simulink model "idle_speed_model_project_pid"  (Simulink 9.1)
settings: Solver=ode45  StartTime=0  StopTime=25  FixedStep=0.01  MaxStep=0.02  RelTol=1e-3  EnableMultiTasking=on
values from neighbouring files (symbols this model uses):
  a = [1.69e-07,-1.136e-06,6.89e-06]    [assign_pid.m]
  gam = 1.35    [assign_pid.m]
  J = 0.0789    [assign_pid.m]
  Kd = 4    [assign_pid.m]
  KI = 0.005    [assign_pid.m]
  KP = 0.8    [assign_pid.m]
  N0 = 828    [assign_pid.m]
  P0 = 26431    [assign_pid.m]
  p_amb = 1.0121*1e5    (= 101210)    [assign_pid.m]
  par_fr = [7.4198e-7 -4.989e-4 11.3]    [assign_pid.m]
  par_IMEP0 = [1.2323e-4 2.1256]    [assign_pid.m]
  par_sp = [-0.0017 -0.0277 1.36]    [assign_pid.m]
  R = 288    [assign_pid.m]
  si = 0.812    [assign_pid.m]
  T_amb = 302    [assign_pid.m]
  Tau_d = pi/3    (= 1.0471975512)    [assign_pid.m]
  Vd = 2.4e-3    (= 0.0024)    [assign_pid.m]
  Vm = 5.8e-3    (= 0.0058)    [assign_pid.m]
  X0 = [26424 21.3765773202354 83.9019428270409]    [assign_pid.m]
  yi = 0.0633    [assign_pid.m]
  Z = 4    [assign_pid.m]
undefined symbols (not defined in the file or in its folder): setp, sigbuilder_block
settings Model: Creator=Canov  LastModifiedBy=VARUN
settings SolverCC: PositivePriorityOrder=on
settings DataIOCC: SignalLoggingSaveFormat=ModelDataLogs  SignalLoggingName=sigsOut
settings OptimizationCC: ExpressionDepthLimit=2147483647  InitFltsAndDblsToZero=on
settings DebuggingCC: SaveWithParameterizedLinksMsg=none  SignalResolutionControl=TryResolveAllWithWarning  MultiTaskDSMMsg=warning  MultiTaskCondExecSysMsg=none  FcnCallInpInsideContextMsg=warning  StateNameClashWarn=warning
settings HardwareCC: TargetBitPerPointer=64  TargetBitPerSizeT=64  TargetBitPerPtrDiffT=64  TargetLongLongMode=on  TargetIntDivRoundTo=Zero  TargetEndianess=LittleEndian  TargetWordSize=64  TargetHWDeviceType=MATLAB Host  ProdEqTarget=off
settings GRTTargetCC: TargetFcnLib=ansi_tfl_tmw.mat  GeneratePreprocessorConditionals=Disable all

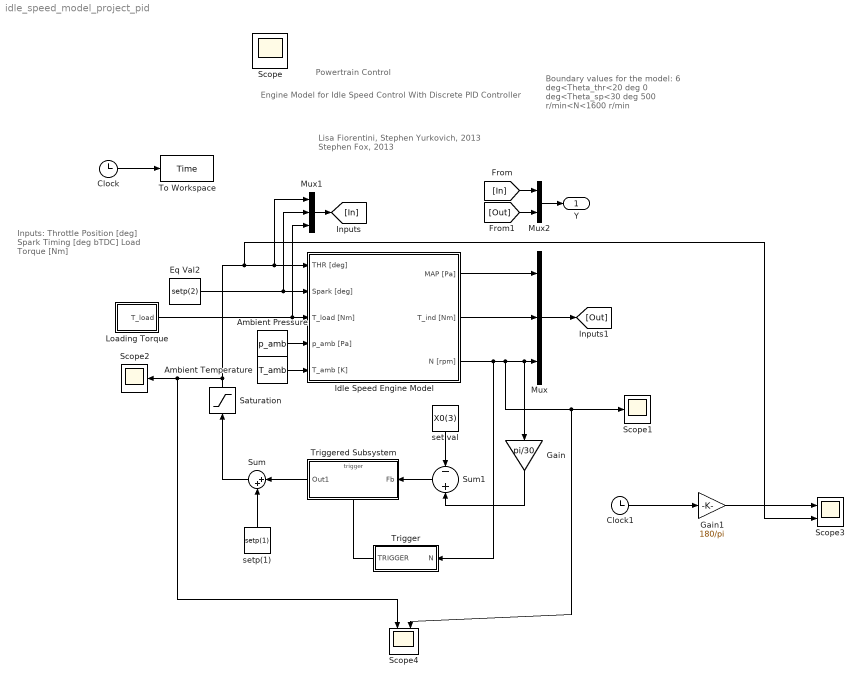
== system idle_speed_model_project_pid ==
  note: Engine Model for Idle Speed Control
      | With Discrete PID Controller
  note: Inputs:
      |
      |
      | Throttle Position [deg]
      |
      | Spark Timing [deg bTDC]
      |
      | Load Torque [Nm]
  note: Powertrain Control
  note: Lisa Fiorentini, Stephen Yurkovich, 2013
      | Stephen Fox, 2013
  note: Boundary values for the model:
      | 6 deg<Theta_thr<20 deg
      | 0 deg<Theta_sp<30 deg
      | 500 r/min<N<1600 r/min
  Ambient Pressure : Constant  Value=p_amb
  Ambient Temperature : Constant  Value=T_amb
  Clock : Clock
  Clock1 : Clock
  Eq Val2 : Constant  Value=setp(2)
  Gain : Gain  Gain=pi/30
  Gain1 : Gain  Gain=180/pi
  Idle Speed Engine Model : Subsystem
  Loading Torque : Subsystem
  Mux : Mux  Inputs=3
  Mux1 : Mux  Inputs=3
  Mux2 : Mux  Inputs=2
  Saturation : Saturate  UpperLimit=20  LowerLimit=6  OutMin=[6]  OutMax=[20]
  Scope1 : Scope
  Scope2 : Scope
  Scope3 : Scope  NumInputPorts=2
  Scope4 : Scope  NumInputPorts=2
  Sum : Sum  Inputs=|++
  Sum1 : Sum  Inputs=-|+
  To Workspace : ToWorkspace  VariableName=Time  SaveFormat=Structure  SampleTime=-1
      settings: Decimation=7  Save2DSignal=2-D array (concatenate along first dimension)
  Trigger : Subsystem
  Triggered Subsystem : Subsystem  TreatAsAtomicUnit=on
  set val : Constant  Value=X0(3)
  setp(1) : Constant  Value=setp(1)
  Y : Outport
  Scope : Scope
  wires:
  Ambient Pressure/1 -> Idle Speed Engine Model/4(p_amb [Pa])
  Ambient Temperature/1 -> Idle Speed Engine Model/5(T_amb [K])
  Eq Val2/1 -> Idle Speed Engine Model/2(Spark [deg]), Mux1/2
  Idle Speed Engine Model/2(T_ind [Nm]) -> Mux/2
  Idle Speed Engine Model/1(MAP [Pa]) -> Mux/1
  Loading Torque/1(T_load) -> Idle Speed Engine Model/3(T_load [Nm]), Mux1/3
  Idle Speed Engine Model/3(N [rpm]) -> Trigger/1(N), Scope4/2, Scope1/1, Mux/3, Gain/1
  Sum/1 -> Saturation/1
  Mux1/1 -> [In]
  Mux/1 -> [Out]
  [In] -> Mux2/1
  [Out] -> Mux2/2
  Mux2/1 -> Y/1
  Triggered Subsystem/1(Out1) -> Sum/1
  setp(1)/1 -> Sum/2
  Gain/1 -> Sum1/2
  Sum1/1 -> Triggered Subsystem/1(Fb)
  set val/1 -> Sum1/1
  Saturation/1 -> Scope4/1, Scope2/1, Scope3/2, Idle Speed Engine Model/1(THR [deg]), Mux1/1
  Trigger/1(TRIGGER) -> Triggered Subsystem/Trigger
  Clock/1 -> To Workspace/1
  Clock1/1 -> Gain1/1
  Gain1/1 -> Scope3/1

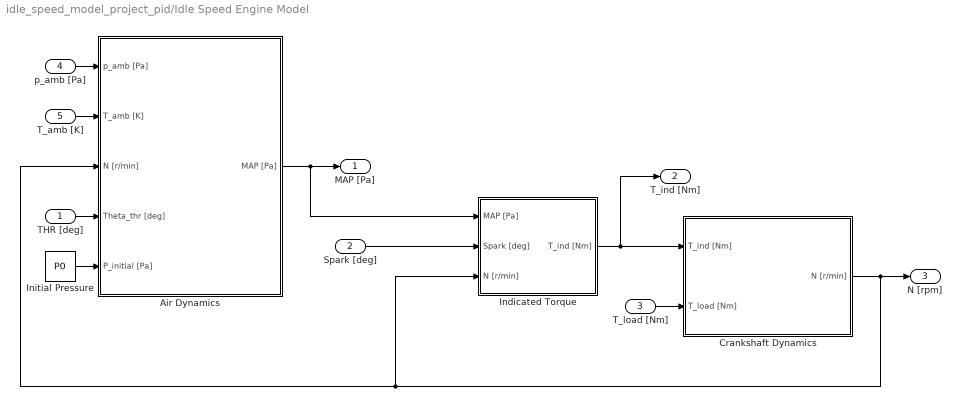
== system idle_speed_model_project_pid/Idle Speed Engine Model ==
  THR [deg] : Inport
  Spark [deg] : Inport  Port=2
  T_load [Nm] : Inport  Port=3
  p_amb [Pa] : Inport  Port=4
  T_amb [K] : Inport  Port=5
  Air Dynamics : Subsystem
  Crankshaft Dynamics : Subsystem
  Indicated Torque : Subsystem
  Initial Pressure : Constant  Value=P0
  MAP [Pa] : Outport
  T_ind [Nm] : Outport  Port=2
  N [rpm] : Outport  Port=3
  wires:
  Spark [deg]/1 -> Indicated Torque/2(Spark [deg])
  Indicated Torque/1(T_ind [Nm]) -> T_ind [Nm]/1, Crankshaft Dynamics/1(T_ind [Nm])
  Air Dynamics/1(MAP [Pa]) -> Indicated Torque/1(MAP [Pa]), MAP [Pa]/1
  Crankshaft Dynamics/1(N [r/min]) -> Indicated Torque/3(N [r/min]), Air Dynamics/3(N [r/min]), N [rpm]/1
  p_amb [Pa]/1 -> Air Dynamics/1(p_amb [Pa])
  T_amb [K]/1 -> Air Dynamics/2(T_amb [K])
  THR [deg]/1 -> Air Dynamics/4(Theta_thr [deg])
  Initial Pressure/1 -> Air Dynamics/5(P_initial [Pa])
  T_load [Nm]/1 -> Crankshaft Dynamics/2(T_load [Nm])

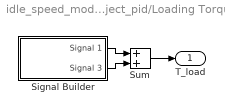
== system idle_speed_model_project_pid/Loading Torque ==
  Signal Builder : Subsystem  Tag=STV Subsys  LoadFcn=sigbuilder_block('load');  StartFcn=sigbuilder_block('start');  StopFcn=sigbuilder_block('stop');  ClipboardFcn=sigbuilder_block('clipboard');  mask(Sigbuilder block){tuvar=[0:10]}
      mask help: Simulink:masks:SigbuilderBlock_MD
      mask init:
      | if ~strcmp(get_param(bdroot(gcbh),'SimulationStatus'),'stopped') tuvar = sigbuilder_block('maskInit'); end
      settings: CopyFcn=sigbuilder_block('copy');  DeleteFcn=sigbuilder_block('delete');  ModelCloseFcn=sigbuilder_block('modelClose');  PreSaveFcn=sigbuilder_block('preSave');  PauseFcn=sigbuilder_block('pause');  ContinueFcn=sigbuilder_block('continue');  NameChangeFcn=sigbuilder_block('namechange');  OpenFcn=sigbuilder_block('open',[6 30 1012.5 447.75 ]);  CloseFcn=sigbuilder_block('close');
      mask Display: plot(0, 0, 100, 100,[2, 2, 32, 32, 2], [68, 8, 8, 68, 68],[32, 2], [38, 38], [32, 19, 2],[53, 60, 44], [32, 17, 17, 2],[16, 16, 31, 31]);txt = getActiveGroup(gcbh);text(2, 100, txt,'verticalAlignment', 'top');
  Sum : Sum
  T_load : Outport
  wires:
  Signal Builder/1(Signal 1) -> Sum/1
  Signal Builder/2(Signal 3) -> Sum/2
  Sum/1 -> T_load/1

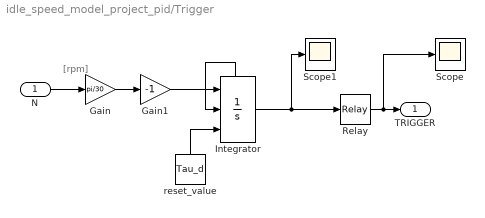
== system idle_speed_model_project_pid/Trigger ==
  note: [rpm]
  N : Inport
  Gain : Gain  Gain=pi/30
  Gain1 : Gain  Gain=-1
  Integrator : Integrator  ExternalReset=falling  InitialConditionSource=external  ShowStatePort=on
  Relay : Relay  OnSwitchValue=0.5*Tau_d  OffSwitchValue=0.5*Tau_d
  Scope : Scope
  Scope1 : Scope
  reset_value : Constant  Value=Tau_d
  TRIGGER : Outport
  wires:
  Relay/1 -> Scope/1, TRIGGER/1
  reset_value/1 -> Integrator/3
  Gain1/1 -> Integrator/1
  Integrator/State -> Integrator/2
  N/1 -> Gain/1
  Gain/1 -> Gain1/1
  Integrator/1 -> Scope1/1, Relay/1

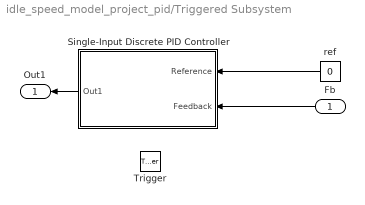
== system idle_speed_model_project_pid/Triggered Subsystem ==
  Fb : Inport
  Trigger : TriggerPort  VariantControl=Variant  PortDimensions=1
  Single-Input Discrete PID Controller : Subsystem
  ref : Constant  Value=0
  Out1 : Outport
  wires:
  ref/1 -> Single-Input Discrete PID Controller/1(Reference)
  Single-Input Discrete PID Controller/1(Out1) -> Out1/1
  Fb/1 -> Single-Input Discrete PID Controller/2(Feedback)

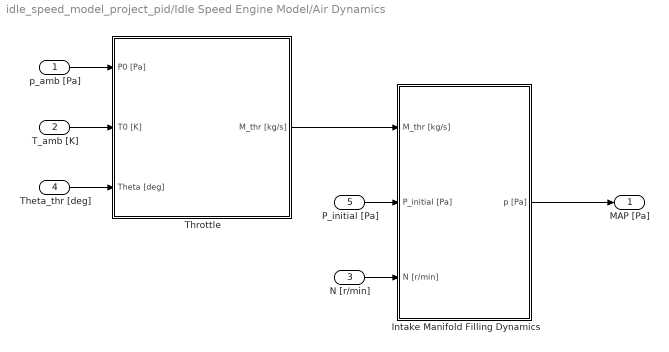
== system idle_speed_model_project_pid/Idle Speed Engine Model/Air Dynamics ==
  p_amb [Pa] : Inport
  T_amb [K] : Inport  Port=2
  N [r/min] : Inport  Port=3
  Theta_thr [deg] : Inport  Port=4
  P_initial [Pa] : Inport  Port=5
  Intake Manifold Filling Dynamics : Subsystem
  Throttle : Subsystem
  MAP [Pa] : Outport
  wires:
  Intake Manifold Filling Dynamics/1(p [Pa]) -> MAP [Pa]/1
  P_initial [Pa]/1 -> Intake Manifold Filling Dynamics/2(P_initial [Pa])
  p_amb [Pa]/1 -> Throttle/1(P0 [Pa])
  T_amb [K]/1 -> Throttle/2(T0 [K])
  Theta_thr [deg]/1 -> Throttle/3(Theta [deg])
  Throttle/1(M_thr [kg/s]) -> Intake Manifold Filling Dynamics/1(M_thr [kg/s])
  N [r/min]/1 -> Intake Manifold Filling Dynamics/3(N [r/min])

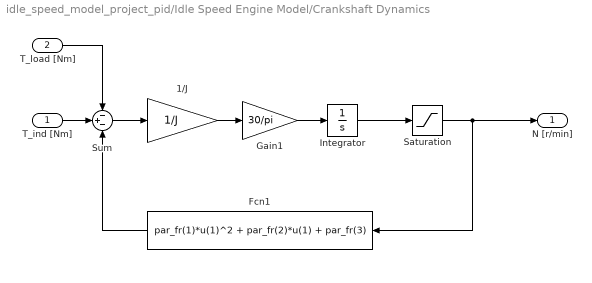
== system idle_speed_model_project_pid/Idle Speed Engine Model/Crankshaft Dynamics ==
  T_ind [Nm] : Inport
  T_load [Nm] : Inport  Port=2
  1/J : Gain  Gain=1/J  SaturateOnIntegerOverflow=on  OutDataTypeStr=Inherit: Same as input  ParamDataTypeStr=Inherit: Same as input
  Fcn1 : Fcn  Expr=par_fr(1)*u(1)^2 + par_fr(2)*u(1) + par_fr(3)
  Gain1 : Gain  Gain=30/pi  SaturateOnIntegerOverflow=on  OutDataTypeStr=Inherit: Same as input  ParamDataTypeStr=Inherit: Same as input
  Integrator : Integrator  InitialCondition=N0
  Saturation : Saturate  UpperLimit=6000  LowerLimit=100
  Sum : Sum  Inputs=-+-  SaturateOnIntegerOverflow=on
  N [r/min] : Outport
  wires:
  Saturation/1 -> N [r/min]/1, Fcn1/1
  T_ind [Nm]/1 -> Sum/2
  T_load [Nm]/1 -> Sum/1
  Sum/1 -> 1/J/1
  1/J/1 -> Gain1/1
  Gain1/1 -> Integrator/1
  Integrator/1 -> Saturation/1
  Fcn1/1 -> Sum/3

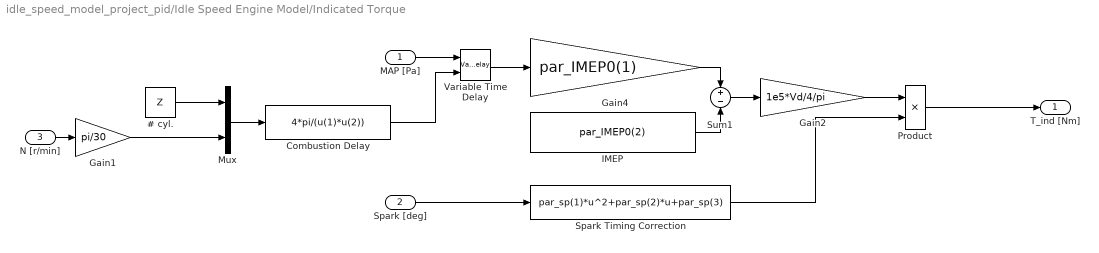
== system idle_speed_model_project_pid/Idle Speed Engine Model/Indicated Torque ==
  MAP [Pa] : Inport
  Spark [deg] : Inport  Port=2
  N [r/min] : Inport  Port=3
  # cyl. : Constant  Value=Z
  Combustion Delay : Fcn  Expr=4*pi/(u(1)*u(2))
  Gain1 : Gain  Gain=pi/30  SaturateOnIntegerOverflow=on  OutDataTypeStr=Inherit: Same as input  ParamDataTypeStr=Inherit: Same as input
  Gain2 : Gain  Gain=1e5*Vd/4/pi  SaturateOnIntegerOverflow=on  OutDataTypeStr=Inherit: Same as input  ParamDataTypeStr=Inherit: Same as input
  Gain4 : Gain  Gain=par_IMEP0(1)  SaturateOnIntegerOverflow=on  OutDataTypeStr=Inherit: Same as input  ParamDataTypeStr=Inherit: Same as input
  IMEP : Constant  Value=par_IMEP0(2)
  Mux : Mux  Inputs=2
  Product : Product  RndMeth=Zero
  Spark Timing Correction : Fcn  Expr=par_sp(1)*u^2+par_sp(2)*u+par_sp(3)
  Sum1 : Sum  Inputs=+-  SaturateOnIntegerOverflow=on
  Variable Time Delay : VariableTransportDelay  InitialOutput=P0  ZeroDelay=on
  T_ind [Nm] : Outport
  wires:
  Spark Timing Correction/1 -> Product/2
  Spark [deg]/1 -> Spark Timing Correction/1
  Gain2/1 -> Product/1
  Gain1/1 -> Mux/2
  Mux/1 -> Combustion Delay/1
  # cyl./1 -> Mux/1
  N [r/min]/1 -> Gain1/1
  Product/1 -> T_ind [Nm]/1
  Gain4/1 -> Sum1/1
  IMEP/1 -> Sum1/2
  Sum1/1 -> Gain2/1
  Combustion Delay/1 -> Variable Time Delay/2
  MAP [Pa]/1 -> Variable Time Delay/1
  Variable Time Delay/1 -> Gain4/1

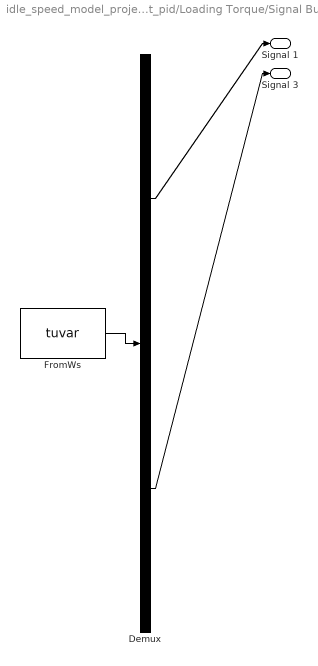
== system idle_speed_model_project_pid/Loading Torque/Signal Builder ==
  Demux : Demux  Tag=STV Demux  Outputs=2
  FromWs : FromWorkspace  Tag=STV FromWs  VariableName=tuvar  SampleTime=0  SigBuilderData=DataTag0  VnvData=DataTag1
      SigBuilderData=|
      | common.afterFinalStr = 'Extrapolate'
      | common.sampleTime = 0
      | dataSet.timeRange = [0 2000]
      | dataSet.name = 'Group 1'
      | sbobj.Groups.Name = 'Group 1'
      | sbobj.Groups.Signals(1).Name = 'Signal 1'
      | sbobj.Groups.Signals(1).XData = [0 5 5 10 10 2000]
      | sbobj.Groups.Signals(1).YData = [10 10 20 20 10 10]
      | sbobj.Groups.Signals(2).Name = 'Signal 3'
      | sbobj.Groups.Signals(2).XData = [0 15 15 20 20 2000]
      | sbobj.Groups.Signals(2).YData = [0 0 -10 -10 0 0]
      | sbobj.Groups.TimeRange = [0 2000]
  Signal 1 : Outport  Tag=STV Outport
  Signal 3 : Outport  Tag=STV Outport  Port=2
  wires:
  FromWs/1 -> Demux/1
  Demux/1 -> Signal 1/1
  Demux/2 -> Signal 3/1

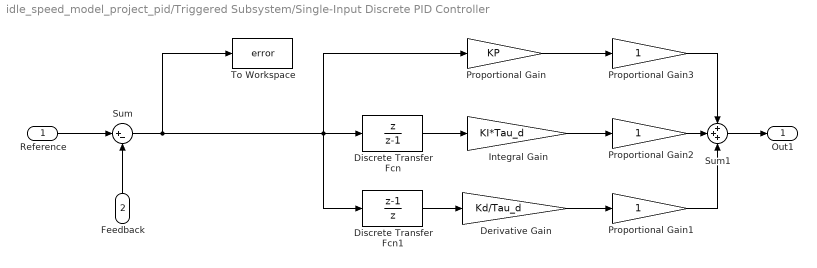
== system idle_speed_model_project_pid/Triggered Subsystem/Single-Input Discrete PID Controller ==
  Reference : Inport
  Feedback : Inport  Port=2
  Derivative Gain : Gain  Gain=Kd/Tau_d
  Discrete Transfer Fcn : DiscreteTransferFcn  Numerator=[1 0]  Denominator=[1 -1]
  Discrete Transfer Fcn1 : DiscreteTransferFcn  Numerator=[1 -1]  Denominator=[1 0]
  Integral Gain : Gain  Gain=KI*Tau_d
  Proportional Gain : Gain  Gain=KP
  Proportional Gain1 : Gain
  Proportional Gain2 : Gain
  Proportional Gain3 : Gain
  Sum : Sum  Inputs=|+-
  Sum1 : Sum  Inputs=+++
  To Workspace : ToWorkspace  VariableName=error  SaveFormat=Structure With Time  SampleTime=-1
      settings: Save2DSignal=2-D array (concatenate along first dimension)
  Out1 : Outport
  wires:
  Discrete Transfer Fcn1/1 -> Derivative Gain/1
  Discrete Transfer Fcn/1 -> Integral Gain/1
  Reference/1 -> Sum/1
  Feedback/1 -> Sum/2
  Proportional Gain/1 -> Proportional Gain3/1
  Integral Gain/1 -> Proportional Gain2/1
  Derivative Gain/1 -> Proportional Gain1/1
  Proportional Gain3/1 -> Sum1/1
  Proportional Gain2/1 -> Sum1/2
  Proportional Gain1/1 -> Sum1/3
  Sum1/1 -> Out1/1
  Sum/1 -> To Workspace/1, Discrete Transfer Fcn1/1, Proportional Gain/1, Discrete Transfer Fcn/1

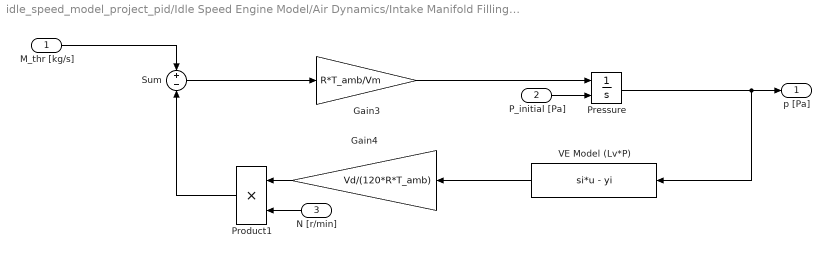
== system idle_speed_model_project_pid/Idle Speed Engine Model/Air Dynamics/Intake Manifold Filling Dynamics ==
  M_thr [kg/s] : Inport
  P_initial [Pa] : Inport  Port=2
  N [r/min] : Inport  Port=3
  Gain3 : Gain  Gain=R*T_amb/Vm  SaturateOnIntegerOverflow=on  OutDataTypeStr=Inherit: Same as input  ParamDataTypeStr=Inherit: Same as input
  Gain4 : Gain  Gain=Vd/(120*R*T_amb)  SaturateOnIntegerOverflow=on  OutDataTypeStr=Inherit: Same as input  ParamDataTypeStr=Inherit: Same as input
  Pressure : Integrator  InitialConditionSource=external
  Product1 : Product  Inputs=**  SaturateOnIntegerOverflow=on  OutDataTypeStr=Inherit: Same as first input
  Sum : Sum  Inputs=+-  SaturateOnIntegerOverflow=on
  VE Model (Lv*P) : Fcn  Expr=si*u - yi
  p [Pa] : Outport
  wires:
  Pressure/1 -> p [Pa]/1, VE Model (Lv*P)/1
  VE Model (Lv*P)/1 -> Gain4/1
  Gain3/1 -> Pressure/1
  P_initial [Pa]/1 -> Pressure/2
  M_thr [kg/s]/1 -> Sum/1
  Sum/1 -> Gain3/1
  Gain4/1 -> Product1/1
  N [r/min]/1 -> Product1/2
  Product1/1 -> Sum/2

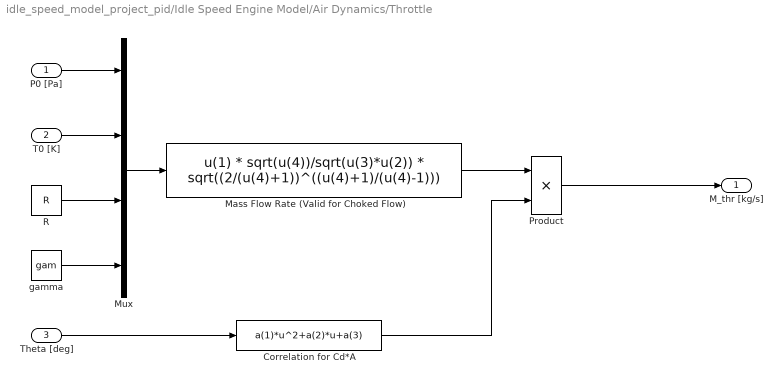
== system idle_speed_model_project_pid/Idle Speed Engine Model/Air Dynamics/Throttle ==
  P0 [Pa] : Inport
  T0 [K] : Inport  Port=2
  Theta [deg] : Inport  Port=3
  Correlation for Cd*A : Fcn  Expr=a(1)*u^2+a(2)*u+a(3)
  Mass Flow Rate (Valid for Choked Flow) : Fcn  Expr=u(1) * sqrt(u(4))/sqrt(u(3)*u(2)) * sqrt((2/(u(4)+1))^((u(4)+1)/(u(4)-1)))
  Mux : Mux
  Product : Product  SaturateOnIntegerOverflow=on  OutDataTypeStr=Inherit: Same as first input
  R : Constant  Value=R
  gamma : Constant  Value=gam
  M_thr [kg/s] : Outport
  wires:
  Correlation for Cd*A/1 -> Product/2
  Theta [deg]/1 -> Correlation for Cd*A/1
  Mass Flow Rate (Valid for Choked Flow)/1 -> Product/1
  P0 [Pa]/1 -> Mux/1
  T0 [K]/1 -> Mux/2
  R/1 -> Mux/3
  gamma/1 -> Mux/4
  Mux/1 -> Mass Flow Rate (Valid for Choked Flow)/1
  Product/1 -> M_thr [kg/s]/1
